simulink model "kalman_filter_adaptive"  (R2020b)
settings: Solver=VariableStepAuto  StartTime=0.0  StopTime=10.0  RelTol=1e-3
values from neighbouring files (symbols this model uses):
  A_d = sys_d.A    [sample_ss.m]
  B_d = sys_d.B    [sample_ss.m]
  C_d = sys_d.C    [sample_ss.m]
  dT = 0.05    [sample_ss.m]
  G = eye(6)    [sample_ss.m]
  Qcov = diag(0.15*ones(1,size(A_m,1)))    [sample_ss.m]
  Rcov = diag(0.05*ones(1,size(A_m,1)))    [sample_ss.m]
undefined symbols (not defined in the file or in its folder): L
libraries: simulink x2
settings Model: Creator=surya  LastModifiedBy=surya

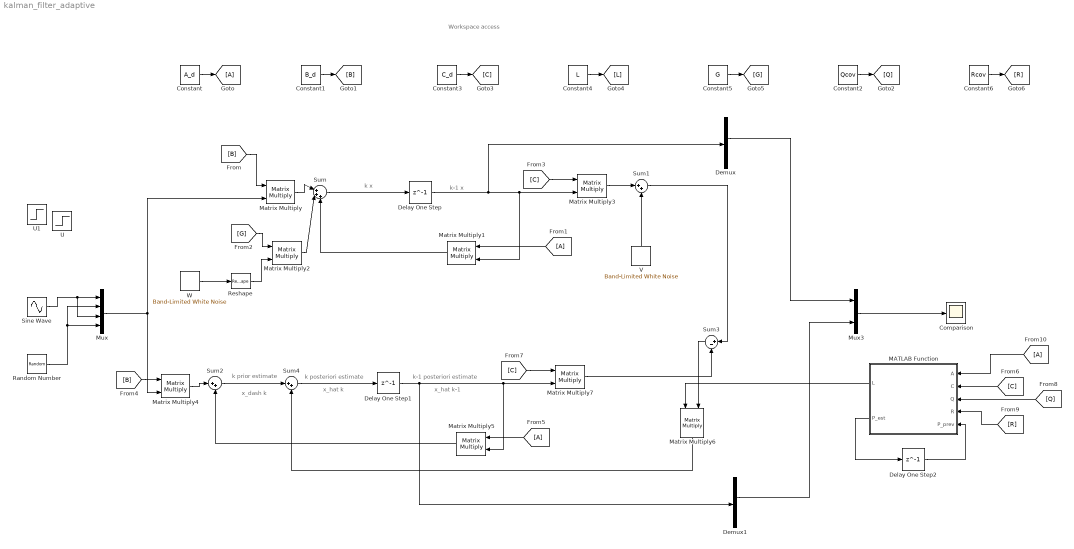
== system kalman_filter_adaptive ==
  note: x_dash k
  note: k prior estimate
  note: x_hat k
  note: k posteriori estimate
  note: k x
  note: x_hat k-1
  note: k-1 x
  note: Workspace access
  note: k-1 posteriori estimate
  Comparison : Scope
  Constant : Constant  Value=A_d
  Constant1 : Constant  Value=B_d
  Constant2 : Constant  Value=Qcov
  Constant3 : Constant  Value=C_d
  Constant4 : Constant  Value=L
  Constant5 : Constant  Value=G
  Constant6 : Constant  Value=Rcov
  Delay One Step : Delay  DelayLength=1  SampleTime=dT
  Delay One Step1 : Delay  DelayLength=1  SampleTime=dT
  Delay One Step2 : Delay  DelayLength=1  InitialCondition=zeros(length(A_d), length(A_d))  SampleTime=dT
  Demux : Demux  Outputs=length(A_d)
  Demux1 : Demux  Outputs=length(A_d)
  MATLAB Function : MATLAB Function  TreatAsAtomicUnit=on
  Matrix Multiply{,1..7} (8 alike) : Product  Multiplication=Matrix(*)
  Mux : Mux
  Mux3 : Mux  Inputs=2
  Random Number : RandomNumber  Variance=10  SampleTime=0.1
  Reshape : Reshape  OutputDimensionality=Customize  OutputDimensions=[length(G(1,:)),1]
  Sine Wave : Sin  SampleTime=0
  Sum : Sum  Inputs=|+++
  Sum1 : Sum  Inputs=|++
  Sum2 : Sum  Inputs=|++
  Sum3 : Sum  Inputs=|+-
  Sum4 : Sum  Inputs=|++
  U : Step  SampleTime=0
  U1 : Step  After=1/2  SampleTime=0
  V : simulink/Sources/Band-Limited White Noise  Cov=[Rcov(1)*dT Rcov(1)*dT Rcov(1)*dT Rcov(1)*dT Rcov(1)*dT Rcov(1)*dT]  Ts=dT  seed=[23341]
  W : simulink/Sources/Band-Limited White Noise  Cov=[Qcov(1)*dT Qcov(1)*dT Qcov(1)*dT Qcov(1)*dT Qcov(1)*dT Qcov(1)*dT]  Ts=dT  seed=[23341]
  wires:
  Demux/3 -> Mux3/1
  V/1 -> Sum1/2
  Matrix Multiply/1 -> Sum/1
  Sum3/1 -> Matrix Multiply6/2
  Matrix Multiply3/1 -> Sum1/1
  [G] -> Matrix Multiply2/1
  [C] -> Matrix Multiply7/1
  [A] -> Matrix Multiply1/1
  Mux3/1 -> Comparison/1
  [A] -> Matrix Multiply5/1
  Matrix Multiply2/1 -> Sum/2
  Delay One Step/1 -> Demux/1, Matrix Multiply1/2, Matrix Multiply3/2
  Mux/1 -> Matrix Multiply4/2, Matrix Multiply/2
  Constant4/1 -> [L]
  Demux1/3 -> Mux3/2
  [B] -> Matrix Multiply/1
  Matrix Multiply1/1 -> Sum/3
  Delay One Step1/1 -> Demux1/1, Matrix Multiply5/2, Matrix Multiply7/2
  Matrix Multiply4/1 -> Sum2/1
  [B] -> Matrix Multiply4/1
  W/1 -> Reshape/1
  Sum/1 -> Delay One Step/1
  Reshape/1 -> Matrix Multiply2/2
  Matrix Multiply5/1 -> Sum2/2
  Matrix Multiply7/1 -> Sum3/2
  Sum1/1 -> Sum3/1
  Constant1/1 -> [B]
  MATLAB Function/1(L) -> Matrix Multiply6/1
  Constant5/1 -> [G]
  [C] -> Matrix Multiply3/1
  Constant3/1 -> [C]
  Constant/1 -> [A]
  Sum2/1 -> Sum4/1
  Sum4/1 -> Delay One Step1/1
  Matrix Multiply6/1 -> Sum4/2
  Delay One Step2/1 -> MATLAB Function/5(P_prev)
  MATLAB Function/2(P_est) -> Delay One Step2/1
  [R] -> MATLAB Function/4(R)
  [Q] -> MATLAB Function/3(Q)
  [C] -> MATLAB Function/2(C)
  [A] -> MATLAB Function/1(A)
  Constant2/1 -> [Q]
  Constant6/1 -> [R]
  Sine Wave/1 -> Mux/3, Mux/1
  Random Number/1 -> Mux/4, Mux/2

== matlab function kalman_filter_adaptive/MATLAB Function ==
  data: A input; C input; Q input; R input; L output; P_prev input; P_est output
function [L, P_est] = fcn(A, C, Q, R, P_prev)

% Prediction
 P_prior = A*P_prev*A' + Q;
 
 % Update
 L = (P_prior*C')*inv(C*P_prior*C' + R);
 P_est = (eye(length(A)) - L*C)*P_prior;
